simulink model "circ_traj_follower"  (R2023b)
settings: Solver=FixedStepAuto  StartTime=0.0  StopTime=10.0  RelTol=1e-3
values from neighbouring files (symbols this model uses):
  leader_inertia = 0.166667    [gazebo.m]
undefined symbols (not defined in the file or in its folder): force, torque
libraries: ros2lib x3, simulink x1, dspsigops x1
settings Model: Creator=matteociviero  LastModifiedBy=matteociviero

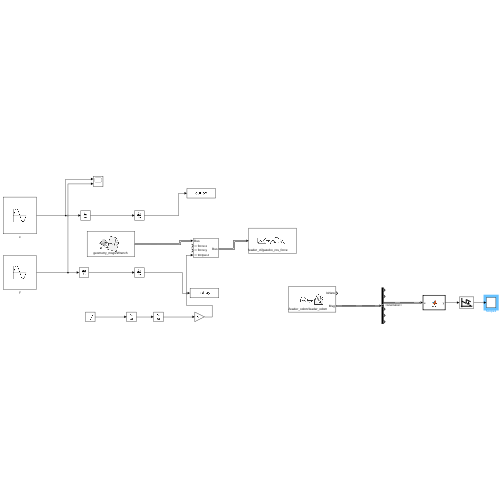
[thumbnail: Simulink's stored preview of the top-level diagram]
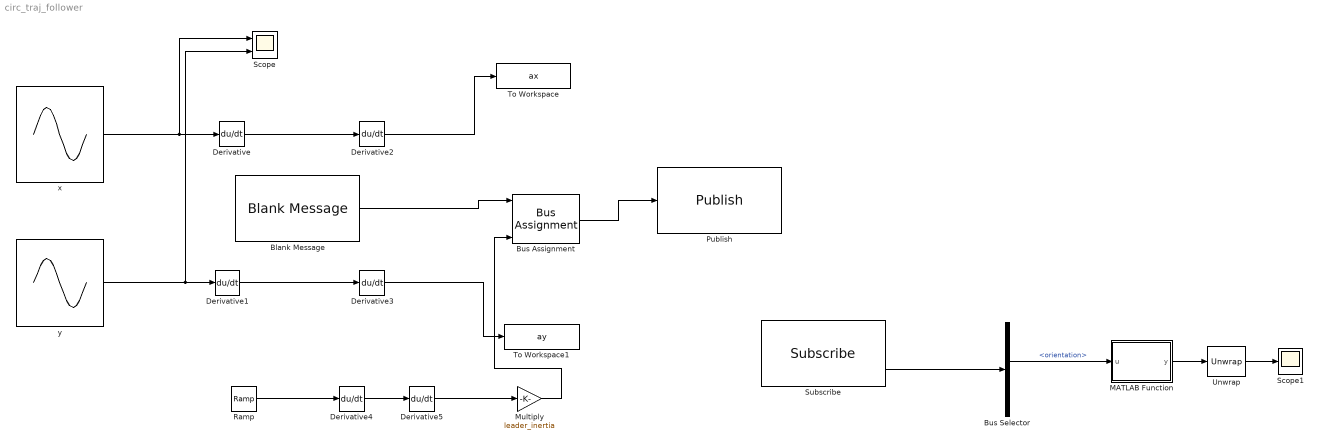
== system circ_traj_follower ==
  Blank Message : ros2lib/Blank Message  messageClass=Message  entityType=geometry_msgs/Wrench  messageType=geometry_msgs/Wrench  SampleTime=0.01
  Bus Assignment : BusAssignment  AssignedSignals=force.x,force.y,torque.z
  Bus Selector : BusSelector  OutputSignals=pose.pose.position.x,pose.pose.position.y,pose.pose.orientation,twist.twist.linear.x,twist.twist.linear.y,twist.twist.angular.z
  Derivative{,1..5} (6 alike) : Derivative
  MATLAB Function : MATLAB Function  TreatAsAtomicUnit=on
  Multiply : Gain  Gain=leader_inertia
  Publish : ros2lib/Publish  topicSource=Select from ROS network  topic=/leader_cf/gazebo_ros_force  messageType=geometry_msgs/Wrench  QOSHistory=Keep last  QOSDepth=1  QOSReliability=Reliable  QOSDurability=Volatile
  Ramp : simulink/Sources/Ramp  slope=2*pi/10  start=0  InitialOutput=0
  Scope : Scope  NumInputPorts=2
  Scope1 : Scope
  Subscribe : ros2lib/Subscribe  topicSource=Select from ROS network  topic=/leader_odom/leader_odom  messageType=nav_msgs/Odometry  sampleTime=-1  QOSHistory=Keep last  QOSDepth=1  QOSReliability=Reliable  QOSDurability=Volatile
  To Workspace : ToWorkspace  VariableName=ax  SaveFormat=Structure With Time  SampleTime=0.01
  To Workspace1 : ToWorkspace  VariableName=ay  SaveFormat=Structure With Time  SampleTime=0.01
  Unwrap : dspsigops/Unwrap  tol=pi  InputProcessing=Columns as channels (frame based)  running=off
  x : Sin  Frequency=2*pi/10  SampleTime=0
  y : Sin  Frequency=2*pi/10  Phase=pi/2  SampleTime=0
  wires:
  x/1 -> Scope/1, Derivative/1
  y/1 -> Scope/2, Derivative1/1
  Derivative/1 -> Derivative2/1
  Derivative1/1 -> Derivative3/1
  Blank Message/1 -> Bus Assignment/1
  Bus Assignment/1 -> Publish/1
  Derivative2/1 -> To Workspace/1
  Derivative3/1 -> To Workspace1/1
  Derivative4/1 -> Derivative5/1
  Derivative5/1 -> Multiply/1
  Multiply/1 -> Bus Assignment/4
  Ramp/1 -> Derivative4/1
  Subscribe/2 -> Bus Selector/1
  Bus Selector/3 -> MATLAB Function/1(u)  "<orientation>"
  MATLAB Function/1(y) -> Unwrap/1
  Unwrap/1 -> Scope1/1

== matlab function circ_traj_follower/MATLAB Function ==
  data: u input; y output
function y = fcn(u)

q = quaternion(u.x, u.y, u.z, u.w);
angles = quat2eul(q);

y = angles(3);
